simulink model "Motorcontrol_Fix"  (R2025b)
settings: Solver=VariableStepAuto  StartTime=0.0  StopTime=5  RelTol=1e-3
values from neighbouring files (symbols this model uses):
  K_motor = K_aug(1:n)    [design_motor_lqr.m]
  Ki_motor = K_aug(n+1)    [design_motor_lqr.m]
  Nbar_motor = rscale_discrete(A, B, C, D, K_motor)    [design_motor_lqr.m]
undefined symbols (not defined in the file or in its folder): A, B, C, DiscIntNeverNeededParam
settings Model: Creator=kenom  LastModifiedBy=MATEO

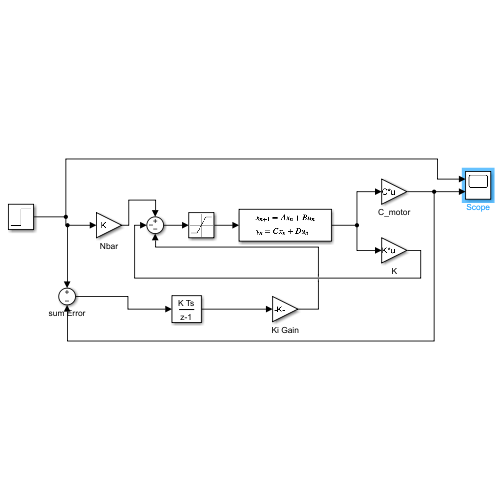
[thumbnail: Simulink's stored preview of the top-level diagram]
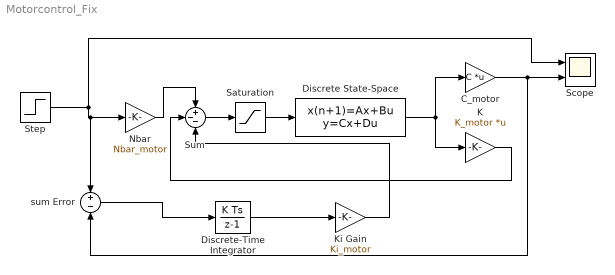
== system Motorcontrol_Fix ==
  C_motor : Gain  Gain=C  Multiplication=Matrix(K*u)
  Discrete State-Space : DiscreteStateSpace  A=A  B=B  C=eye(size(A))  D=zeros(size(A,1),1)  SampleTime=0.1
  Discrete-Time Integrator : DiscreteIntegrator  SampleTime=0.1  ICPrevOutput=DiscIntNeverNeededParam  ICPrevScaledInput=DiscIntNeverNeededParam
  K : Gain  Gain=K_motor  Multiplication=Matrix(K*u)
  Ki Gain : Gain  Gain=Ki_motor
  Nbar : Gain  Gain=Nbar_motor
  Saturation : Saturate  UpperLimit=255  LowerLimit=-255
  Scope : Scope  NumInputPorts=2
      settings: ActiveDisplayYMinimum=-144035.88275616037  ActiveDisplayYMaximum=2852.4700475237596
  Step : Step  Time=0  After=28  SampleTime=0.1
  Sum : Sum  Inputs=+--
  sum Error : Sum  Inputs=+-
  wires:
  Nbar/1 -> Sum/1
  Sum/1 -> Saturation/1
  Saturation/1 -> Discrete State-Space/1
  K/1 -> Sum/2
  Step/1 -> sum Error/1, Nbar/1, Scope/1
  Discrete State-Space/1 -> C_motor/1, K/1
  C_motor/1 -> Scope/2, sum Error/2
  sum Error/1 -> Discrete-Time Integrator/1
  Discrete-Time Integrator/1 -> Ki Gain/1
  Ki Gain/1 -> Sum/3
